simulink model "DPT"  (R2023a)
settings: Solver=VariableStepAuto  StartTime=0.0  StopTime=25  RelTol=1e-3
values from neighbouring files (symbols this model uses):
  beta = 0.001    [main.m]
  C_m = 1.3    [main.m]
  C_w = 3.15    [main.m]
  J_dv = 7 * 10^-6    (= 7e-06)    [main.m]
  L_a = 0.0015    [main.m]
  L_ov = 0.013    [main.m]
  R_a = 8    [main.m]
settings Model: Creator=ycheb  LastModifiedBy=ycheb

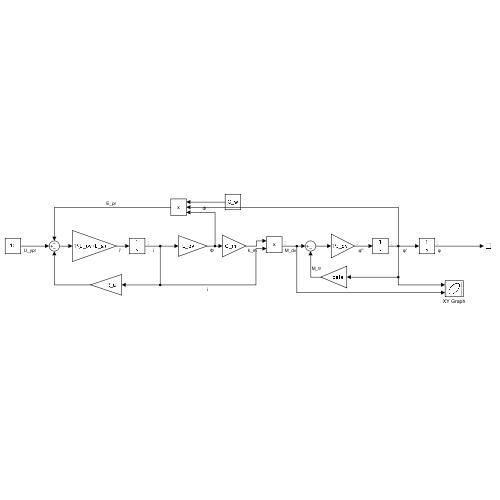
[thumbnail: Simulink's stored preview of the top-level diagram]
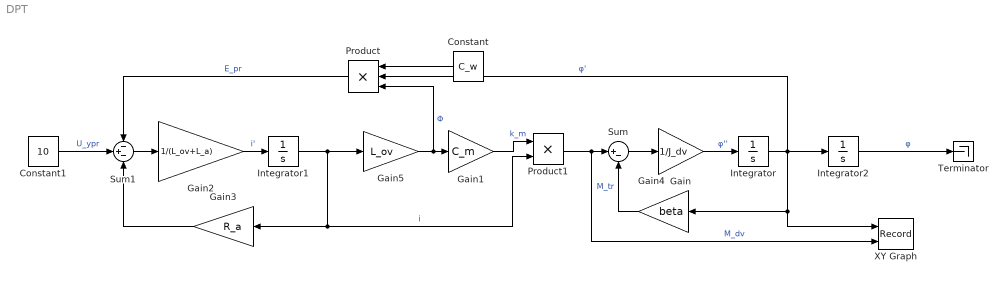
== system DPT ==
  Constant : Constant  Value=C_w
  Constant1 : Constant  Value=10
  Gain : Gain  Gain=1/J_dv
  Gain1 : Gain  Gain=C_m
  Gain2 : Gain  Gain=1/(L_ov+L_a)
  Gain3 : Gain  Gain=R_a
  Gain4 : Gain  Gain=beta
  Gain5 : Gain  Gain=L_ov
  Integrator : Integrator
  Integrator1 : Integrator
  Integrator2 : Integrator
  Product : Product  Inputs=3
  Product1 : Product
  Sum : Sum  Inputs=|+-
  Sum1 : Sum  Inputs=-+-
  Terminator : Terminator
  XY Graph : Record  FileSettingsInternal="{\"entries\":[{\"content\":{\"excelSettings\":{\"content\":{},\"type\":\"Streamout.ExcelSettings\"}},\"type\":\"Streamout.FileSettingStorage\",\"uuid\":\"\"}],\"packageUris\":[\"http:\\/\\/schema.mathworks.com\\/mf0\\/streamout_blocks\\/R2020a\"],\"version\":\"1.0\"}"  Layout=[1 1]  SignalsInternal="{\"entries\":[{\"content\":{\"signals\":[{\"content\":{\"blockPath\":[],\"dimensions\":[1],\"domain\":\"\",\"lineColor\":\"#a2142f\",\"plots\":[1],\"port\":1,\"sid\":[\"\"],\"signalID\":232,\"signalName\":\"φ'\"},\"type\":\"RecordBlkView.Signal\",\"uuid\":\"\"},{\"content\":{\"blockPath\":[],\"dimensions\":[1],\"domain\":\"\",\"lineColor\":\"#139fff\",\"plots\":[1],\"port\":2,\"sid\":[\"\"],\"signalID\":236,\"signalName\":\"M_dv\"},\"type\":\"RecordBlkView.Signal\",\"uuid\":\"\"}]},\"type\":\"RecordBlkView.InputSignals\",\"uuid\":\"\"}],\"packageUris\":[\"http:\\/\\/schema.mathworks.com\\/mf0\\/streamout_blocks\\/R2020a\"],\"version\":\"1.0\"}"  VisualizationBindings="{\"xyplotplugin\":{\"info\":[{\"series\":[{\"bindingParametersList\":[{\"parameter\":\"X-Axis\",\"signalID\":232,\"signalName\":\"φ'\"},{\"parameter\":\"Y-Axis\",\"signalID\":236,\"signalName\":\"M_dv\"}],\"seriesID\":46091}],\"subplotID\":1}]}}"  CompatibilityTag=XY
  wires:
  Integrator/1 -> Gain4/1, XY Graph/1, Product/2, Integrator2/1  "φ'"
  Sum/1 -> Gain/1
  Gain/1 -> Integrator/1  "φ''"
  Integrator1/1 -> Gain5/1, Product1/2, Gain3/1  "i"
  Gain4/1 -> Sum/2  "M_tr"
  Gain2/1 -> Integrator1/1  "i'"
  Sum1/1 -> Gain2/1
  Constant1/1 -> Sum1/2  "U_ypr"
  Gain3/1 -> Sum1/3
  Gain5/1 -> Product/3, Gain1/1  "Φ"
  Product/1 -> Sum1/1  "E_pr"
  Constant/1 -> Product/1
  Integrator2/1 -> Terminator/1  "φ"
  Gain1/1 -> Product1/1  "k_m"
  Product1/1 -> XY Graph/2, Sum/1  "M_dv"
